simulink model "ClosedLoopSys"  (R2025b)
settings: Solver=ode4  StartTime=0.00  StopTime=10  FixedStep=T  RelTol=1e-5  EnableMultiTasking=on
undefined symbols (not defined in the file or in its folder): amp_sat_l, amp_sat_u, DAC_lim_l, DAC_lim_u, Discrete, g, Je, Jp, Jt, k_d, k_fan, k_N, k_s, l, l1, l2, l3, m1, m2, N, nu, nx, Q, q, QN, sys_fan, T, T_mpc, Time, U_e, x0, xfe
libraries: ctrlSharedLib x1
settings Model: Creator=bjones  LastModifiedBy=leeta
settings SolverCC: AlgebraicLoopSolver=TrustRegion
settings DataIOCC: SaveFormat=Array  SignalLoggingSaveFormat=ModelDataLogs  ReturnWorkspaceOutputs=off
settings OptimizationCC: BlockReduction=off  BooleanDataType=off  ExpressionDepthLimit=2147483647.0  LifeSpan=inf
settings DebuggingCC: SaveWithParameterizedLinksMsg=none  MergeDetectMultiDrivingBlocksExec=none  SignalResolutionControl=TryResolveAllWithWarning  MultiTaskDSMMsg=warning  MultiTaskCondExecSysMsg=none  FcnCallInpInsideContextMsg=warning  UnconnectedInputMsg=warning  UnconnectedOutputMsg=warning  UnconnectedLineMsg=warning  StateNameClashWarn=warning  SFUnexpectedBacktrackingDiag=warning  SFNoUnconditionalDefaultTransitionDiag=warning  SFExecutionAtInitializationDiag=none  ArithmeticOperatorsInVariantConditions=warning
settings HardwareCC: ProdBitPerPointer=32.0  ProdBitPerSizeT=32.0  ProdBitPerPtrDiffT=32.0  ProdLargestAtomicFloat=None  ProdIntDivRoundTo=Undefined  ProdEndianess=Unspecified  ProdWordSize=32.0  ProdHWDeviceType=32-bit Generic  TargetUnknown=on
settings ModelReferenceCC: EnableRefExpFcnMdlSchedulingChecks=on  PropagateSignalLabelsOutOfModel=off
settings SFSimCC: SimUseLocalCustomCode=off  CustomCodeUndefinedFunction=UseInterfaceOnly
settings RTWCC: RTWUseLocalCustomCode=off  GPUComputeCapability=3.5
settings CodeAppCC: StateflowObjectComments=on
settings GRTTargetCC: TargetLangStandard=C89/C90 (ANSI)  CombineOutputUpdateFcns=off  GRTInterface=on
settings ConfigComp: CovMetricSettings=dw  CovSaveCumulativeToWorkspaceVar=on  CovSaveSingleToWorkspaceVar=on  CovExternalEMLEnable=off  CovSFcnEnable=off

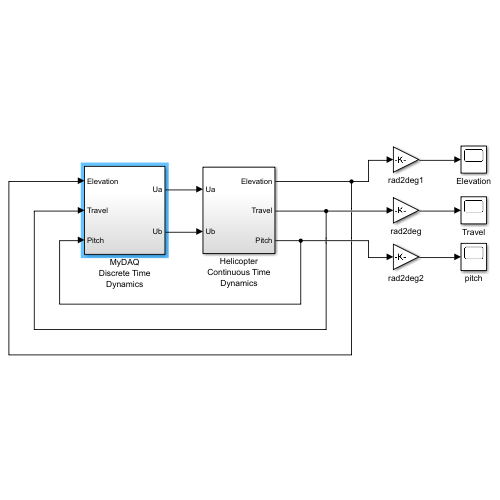
[thumbnail: Simulink's stored preview of the top-level diagram]
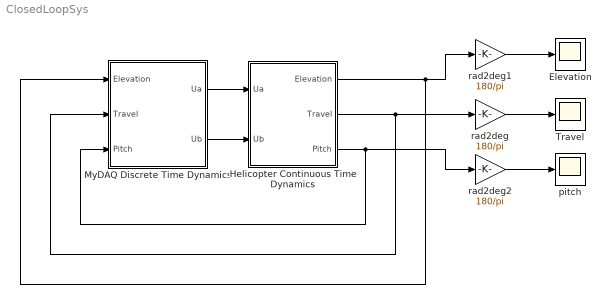
== system ClosedLoopSys ==
  Elevation : Scope
      settings: TimeSpan=60  ActiveDisplayYMinimum=-50  ActiveDisplayYMaximum=30  DataLoggingVariableName=elev
  Helicopter Continuous Time Dynamics : Subsystem
  MyDAQ Discrete Time Dynamics : Subsystem
  Travel : Scope
      settings: TimeSpan=60  ActiveDisplayYMinimum=-150  ActiveDisplayYMaximum=300  DataLoggingVariableName=trav
  pitch : Scope
      settings: TimeSpan=60  ActiveDisplayYMinimum=-25  ActiveDisplayYMaximum=20  DataLoggingVariableName=pitch
  rad2deg : Gain  Gain=180/pi  SaturateOnIntegerOverflow=on  OutDataTypeStr=Inherit: Same as input  ParamDataTypeStr=Inherit: Same as input
  rad2deg1 : Gain  Gain=180/pi  SaturateOnIntegerOverflow=on  OutDataTypeStr=Inherit: Same as input  ParamDataTypeStr=Inherit: Same as input
  rad2deg2 : Gain  Gain=180/pi  SaturateOnIntegerOverflow=on  OutDataTypeStr=Inherit: Same as input  ParamDataTypeStr=Inherit: Same as input
  wires:
  rad2deg/1 -> Travel/1
  rad2deg1/1 -> Elevation/1
  Helicopter Continuous Time Dynamics/2(Travel) -> MyDAQ Discrete Time Dynamics/2(Travel), rad2deg/1
  Helicopter Continuous Time Dynamics/1(Elevation) -> rad2deg1/1, MyDAQ Discrete Time Dynamics/1(Elevation)
  rad2deg2/1 -> pitch/1
  Helicopter Continuous Time Dynamics/3(Pitch) -> rad2deg2/1, MyDAQ Discrete Time Dynamics/3(Pitch)
  MyDAQ Discrete Time Dynamics/1(Ua) -> Helicopter Continuous Time Dynamics/1(Ua)
  MyDAQ Discrete Time Dynamics/2(Ub) -> Helicopter Continuous Time Dynamics/2(Ub)

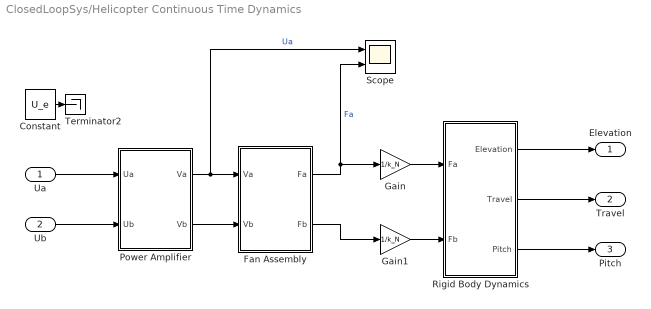
== system ClosedLoopSys/Helicopter Continuous Time Dynamics ==
  Ua : Inport
  Ub : Inport  Port=2
  Constant : Constant  Value=U_e
  Fan Assembly : Subsystem
  Gain : Gain  Gain=1/k_N
  Gain1 : Gain  Gain=1/k_N
  Power Amplifier : Subsystem
  Rigid Body Dynamics : Subsystem
  Scope : Scope  NumInputPorts=2
      settings: ActiveDisplayYMinimum=-1.0960612962914624  ActiveDisplayYMaximum=9.9757218399878962  DataLoggingVariableName=ScopeData5
  Terminator2 : Terminator
  Elevation : Outport
  Travel : Outport  Port=2
  Pitch : Outport  Port=3
  wires:
  Power Amplifier/1(Va) -> Scope/1, Fan Assembly/1(Va)  "Ua"
  Power Amplifier/2(Vb) -> Fan Assembly/2(Vb)
  Rigid Body Dynamics/1(Elevation) -> Elevation/1
  Rigid Body Dynamics/3(Pitch) -> Pitch/1
  Fan Assembly/2(Fb) -> Gain1/1
  Rigid Body Dynamics/2(Travel) -> Travel/1
  Fan Assembly/1(Fa) -> Scope/2, Gain/1  "Fa"
  Ub/1 -> Power Amplifier/2(Ub)
  Constant/1 -> Terminator2/1
  Ua/1 -> Power Amplifier/1(Ua)
  Gain/1 -> Rigid Body Dynamics/1(Fa)
  Gain1/1 -> Rigid Body Dynamics/2(Fb)

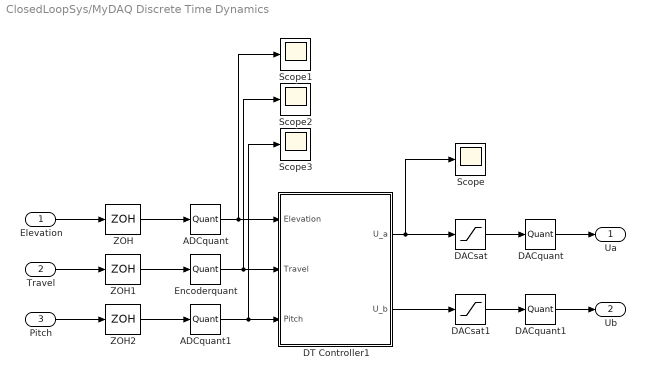
== system ClosedLoopSys/MyDAQ Discrete Time Dynamics ==
  Elevation : Inport
  Travel : Inport  Port=2
  Pitch : Inport  Port=3
  ADCquant : Quantizer  QuantizationInterval=ADC_Vres  SampleTime=T
  ADCquant1 : Quantizer  QuantizationInterval=ADC_Vres  SampleTime=T
  DACquant : Quantizer  QuantizationInterval=DAC_Vres  SampleTime=T
  DACquant1 : Quantizer  QuantizationInterval=DAC_Vres  SampleTime=T
  DACsat : Saturate  UpperLimit=DAC_lim_u  LowerLimit=DAC_lim_l  SampleTime=T
  DACsat1 : Saturate  UpperLimit=DAC_lim_u  LowerLimit=DAC_lim_l  SampleTime=T
  DT Controller1 : Subsystem
  Encoderquant : Quantizer  QuantizationInterval=Encoder_res  SampleTime=T
  Scope{,1..3} (4 alike) : Scope
      Scope settings: ActiveDisplayYMinimum=-1  ActiveDisplayYMaximum=1
      Scope1 settings: ActiveDisplayYMinimum=-0.1017  ActiveDisplayYMaximum=0.78714  DataLoggingVariableName=ScopeData2
      Scope2 settings: ActiveDisplayYMinimum=-1  ActiveDisplayYMaximum=1
      Scope3 settings: ActiveDisplayYMinimum=-1  ActiveDisplayYMaximum=1  DataLoggingVariableName=ScopeData2
  ZOH : ZeroOrderHold  SampleTime=T
  ZOH1 : ZeroOrderHold  SampleTime=T
  ZOH2 : ZeroOrderHold  SampleTime=T
  Ua : Outport
  Ub : Outport  Port=2
  wires:
  Elevation/1 -> ZOH/1
  Travel/1 -> ZOH1/1
  DACquant/1 -> Ua/1
  DACquant1/1 -> Ub/1
  DT Controller1/1(U_a) -> Scope/1, DACsat/1
  DACsat/1 -> DACquant/1
  DT Controller1/2(U_b) -> DACsat1/1
  DACsat1/1 -> DACquant1/1
  ZOH1/1 -> Encoderquant/1
  ZOH/1 -> ADCquant/1
  Pitch/1 -> ZOH2/1
  ZOH2/1 -> ADCquant1/1
  ADCquant/1 -> Scope1/1, DT Controller1/1(Elevation)
  ADCquant1/1 -> Scope3/1, DT Controller1/3(Pitch)
  Encoderquant/1 -> Scope2/1, DT Controller1/2(Travel)

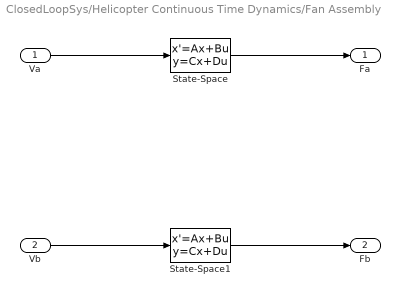
== system ClosedLoopSys/Helicopter Continuous Time Dynamics/Fan Assembly ==
  Va : Inport
  Vb : Inport  Port=2
  State-Space : StateSpace  A=sys_fan.A  B=sys_fan.B  C=sys_fan.C  D=sys_fan.D  InitialCondition=U_e*k_fan
  State-Space1 : StateSpace  A=sys_fan.A  B=sys_fan.B  C=sys_fan.C  D=sys_fan.D  InitialCondition=U_e*k_fan
  Fa : Outport
  Fb : Outport  Port=2
  wires:
  Va/1 -> State-Space/1
  State-Space1/1 -> Fb/1
  Vb/1 -> State-Space1/1
  State-Space/1 -> Fa/1

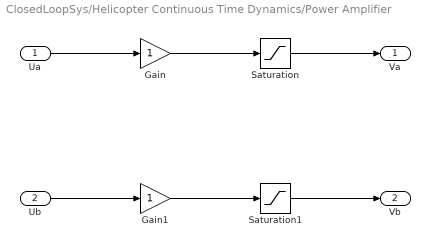
== system ClosedLoopSys/Helicopter Continuous Time Dynamics/Power Amplifier ==
  Ua : Inport
  Ub : Inport  Port=2
  Gain : Gain
  Gain1 : Gain
  Saturation : Saturate  UpperLimit=amp_sat_u  LowerLimit=amp_sat_l
  Saturation1 : Saturate  UpperLimit=amp_sat_u  LowerLimit=amp_sat_l
  Va : Outport
  Vb : Outport  Port=2
  wires:
  Ua/1 -> Gain/1
  Gain/1 -> Saturation/1
  Saturation/1 -> Va/1
  Saturation1/1 -> Vb/1
  Gain1/1 -> Saturation1/1
  Ub/1 -> Gain1/1

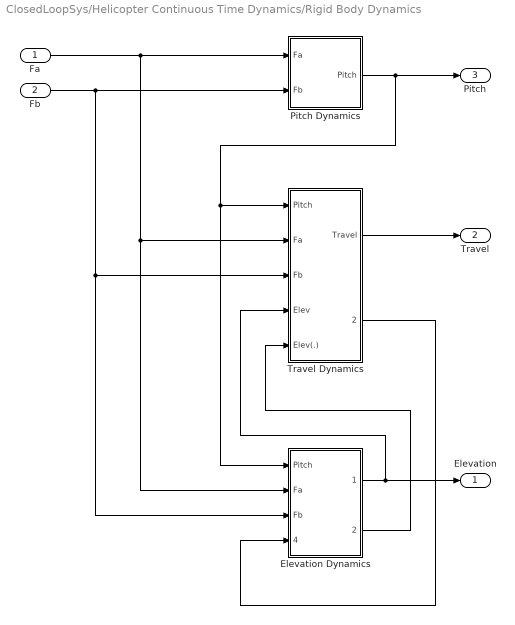
== system ClosedLoopSys/Helicopter Continuous Time Dynamics/Rigid Body Dynamics ==
  Fa : Inport
  Fb : Inport  Port=2
  Elevation Dynamics : Subsystem
  Pitch Dynamics : Subsystem
  Travel Dynamics : Subsystem
  Elevation : Outport
  Travel : Outport  Port=2
  Pitch : Outport  Port=3
  wires:
  Fa/1 -> Pitch Dynamics/1(Fa), Travel Dynamics/2(Fa), Elevation Dynamics/2(Fa)
  Fb/1 -> Pitch Dynamics/2(Fb), Elevation Dynamics/3(Fb), Travel Dynamics/3(Fb)
  Travel Dynamics/1(Travel) -> Travel/1
  Elevation Dynamics/1(Elevation) -> Elevation/1, Travel Dynamics/4(Elev)
  Pitch Dynamics/1(Pitch) -> Travel Dynamics/1(Pitch), Elevation Dynamics/1(Pitch), Pitch/1
  Travel Dynamics/2(Travel(.)) -> Elevation Dynamics/4(Travel(.))
  Elevation Dynamics/2(Elevation(.)) -> Travel Dynamics/5(Elev(.))

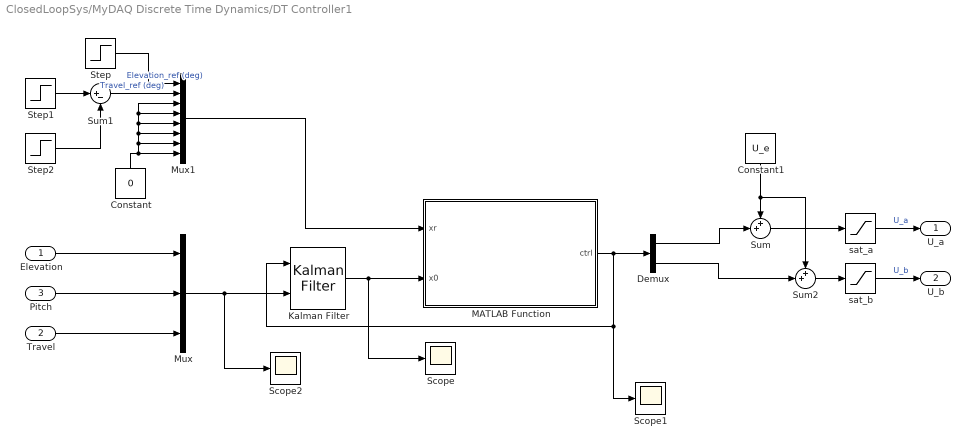
== system ClosedLoopSys/MyDAQ Discrete Time Dynamics/DT Controller1 ==
  Elevation : Inport
  Travel : Inport  Port=2
  Pitch : Inport  Port=3
  Constant : Constant  Value=0
  Constant1 : Constant  Value=U_e
  Demux : Demux  Outputs=2
  Kalman Filter : ctrlSharedLib/Kalman Filter  TimeDomain=Discrete-Time  UseCurrentEstimator=on  ModelSource=LTI State-Space Variable  ModelSourceVariable=sysdt_comb  A=0.95  B=1  C=1  D=0  NumberOfStates=1  NumberOfInputs=1  NumberOfOutputs=1  InitialEstimateSource=Dialog  X0=x0  P0=10  UseK=off  UseGH=off  NumberOfProcessNoiseInputs=1  G=1  TimeInvariantG=on  H=0  TimeInvariantH=on  Q=0.05  TimeInvariantQ=on  R=1  TimeInvariantR=on  N=0  TimeInvariantN=on  AddInputPort=on  AddEnablePort=off  OutputEstimatedY=off  OutputP=off  Ts=-1
  MATLAB Function : MATLAB Function  TreatAsAtomicUnit=on
  Mux : Mux  Inputs=3
  Mux1 : Mux  Inputs=8
  Scope : Scope
      settings: ActiveDisplayYMinimum=-2.4396283803217269  ActiveDisplayYMaximum=1.6155430663981798  DataLoggingVariableName=ScopeData3
  Scope1 : Scope
      settings: ActiveDisplayYMinimum=-1.19057  ActiveDisplayYMaximum=4.48934  DataLoggingVariableName=ScopeData4
  Scope2 : Scope
      settings: ActiveDisplayYMinimum=-0.1017  ActiveDisplayYMaximum=0.78714  DataLoggingVariableName=ScopeData3
  Step : Step  Time=0  Before=x0(1)  After=0  SampleTime=T_mpc
  Step1 : Step  Time=x0(2)  After=0  SampleTime=T_mpc
  Step2 : Step  Time=0  Before=x0(3)  After=0  SampleTime=T_mpc
  Sum : Sum  Inputs=++|
  Sum1 : Sum  Inputs=|+-
  Sum2 : Sum  Inputs=++|
  sat_a : Saturate  UpperLimit=DAC_lim_u  LowerLimit=DAC_lim_l
  sat_b : Saturate  UpperLimit=DAC_lim_u  LowerLimit=DAC_lim_l
  U_a : Outport
  U_b : Outport  Port=2
  wires:
  Step1/1 -> Sum1/1
  Step2/1 -> Sum1/2
  sat_b/1 -> U_b/1  "U_b"
  sat_a/1 -> U_a/1  "U_a"
  Step/1 -> Mux1/1  "Elevation_ref (deg)"
  Sum1/1 -> Mux1/2  "Travel_ref (deg)"
  Elevation/1 -> Mux/1
  Pitch/1 -> Mux/2
  Travel/1 -> Mux/3
  Mux/1 -> Scope2/1, Kalman Filter/2
  Kalman Filter/1 -> Scope/1, MATLAB Function/2(x0)
  MATLAB Function/1(ctrl) -> Scope1/1, Kalman Filter/1, Demux/1
  Constant/1 -> Mux1/8, Mux1/6, Mux1/4, Mux1/3, Mux1/5, Mux1/7
  Mux1/1 -> MATLAB Function/1(xr)
  Demux/1 -> Sum/2
  Demux/2 -> Sum2/2
  Sum/1 -> sat_a/1
  Sum2/1 -> sat_b/1
  Constant1/1 -> Sum2/1, Sum/1

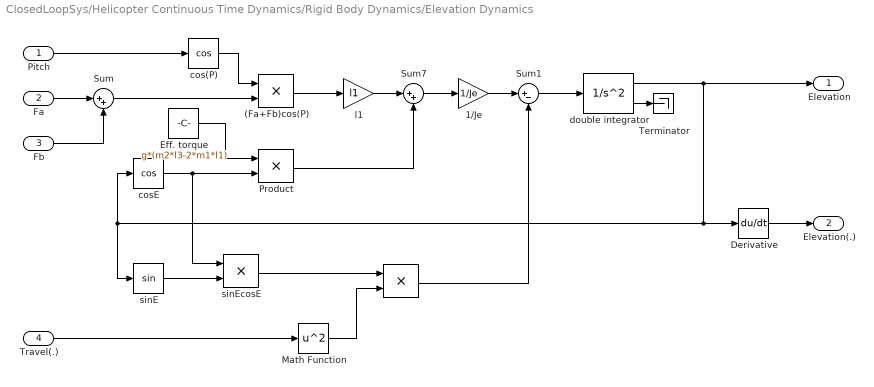
== system ClosedLoopSys/Helicopter Continuous Time Dynamics/Rigid Body Dynamics/Elevation Dynamics ==
  Pitch : Inport
  Fa : Inport  Port=2
  Fb : Inport  Port=3
  Travel(.) : Inport  Port=4
  " " : Product  InputSameDT=on  RndMeth=Zero  SaturateOnIntegerOverflow=on  OutDataTypeStr=Inherit: Same as first input
  (Fa+Fb)cos(P) : Product  InputSameDT=on  RndMeth=Zero  SaturateOnIntegerOverflow=on  OutDataTypeStr=Inherit: Same as first input
  1/Je : Gain  Gain=1/Je  SaturateOnIntegerOverflow=on  OutDataTypeStr=Inherit: Same as input  ParamDataTypeStr=Inherit: Same as input
  Derivative : Derivative
  Eff. torque : Constant  Value=g*(m2*l3-2*m1*l1)
  Math Function : Math  Operator=square  SignedPower=on
  Product : Product  InputSameDT=on  RndMeth=Zero  SaturateOnIntegerOverflow=on  OutDataTypeStr=Inherit: Same as first input
  Sum : Sum  Inputs=|++  InputSameDT=on  SaturateOnIntegerOverflow=on  OutDataTypeStr=Inherit: Same as first input
  Sum1 : Sum  Inputs=|+-  InputSameDT=on  SaturateOnIntegerOverflow=on  OutDataTypeStr=Inherit: Same as first input
  Sum7 : Sum  Inputs=|++  InputSameDT=on  SaturateOnIntegerOverflow=on  OutDataTypeStr=Inherit: Same as first input
  Terminator : Terminator
  cos(P) : Trigonometry  Operator=cos
  cosE : Trigonometry  Operator=cos
  double integrator : SecondOrderIntegrator  ICX=x0(3)  LimitX=on  UpperLimitX=e_lim_u  LowerLimitX=e_lim_l  LimitDXDT=on  UpperLimitDXDT=2*pi  LowerLimitDXDT=-2*pi
  l1 : Gain  Gain=l1  SaturateOnIntegerOverflow=on  OutDataTypeStr=Inherit: Same as input  ParamDataTypeStr=Inherit: Same as input
  sinE : Trigonometry
  sinEcosE : Product  InputSameDT=on  RndMeth=Zero  SaturateOnIntegerOverflow=on  OutDataTypeStr=Inherit: Same as first input
  Elevation : Outport
  Elevation(.) : Outport  Port=2
  wires:
  double integrator/1 -> Elevation/1, sinE/1, cosE/1, Derivative/1
  Derivative/1 -> Elevation(.)/1
  double integrator/2 -> Terminator/1
  Pitch/1 -> cos(P)/1
  Fa/1 -> Sum/1
  Fb/1 -> Sum/2
  cos(P)/1 -> (Fa+Fb)cos(P)/1
  Sum/1 -> (Fa+Fb)cos(P)/2
  (Fa+Fb)cos(P)/1 -> l1/1
  l1/1 -> Sum7/1
  Sum7/1 -> 1/Je/1
  1/Je/1 -> Sum1/1
  Sum1/1 -> double integrator/1
  Travel(.)/1 -> Math Function/1
  Eff. torque/1 -> Product/1
  cosE/1 -> sinEcosE/1, Product/2
  sinE/1 -> sinEcosE/2
  sinEcosE/1 -> " "/1
  Math Function/1 -> " "/2
  Product/1 -> Sum7/2
  " "/1 -> Sum1/2

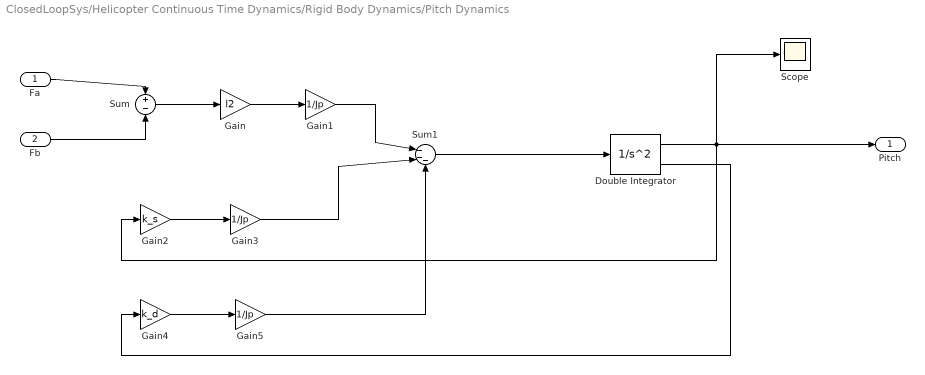
== system ClosedLoopSys/Helicopter Continuous Time Dynamics/Rigid Body Dynamics/Pitch Dynamics ==
  Fa : Inport
  Fb : Inport  Port=2
  Double Integrator : SecondOrderIntegrator  ICX=x0(1)  LimitX=on  UpperLimitX=p_lim_u  LowerLimitX=p_lim_l
  Gain : Gain  Gain=l2
  Gain1 : Gain  Gain=1/Jp
  Gain2 : Gain  Gain=k_s
  Gain3 : Gain  Gain=1/Jp
  Gain4 : Gain  Gain=k_d
  Gain5 : Gain  Gain=1/Jp
  Scope : Scope
      settings: ActiveDisplayYMinimum=-1  ActiveDisplayYMaximum=1  DataLoggingVariableName=ScopeData2
  Sum : Sum  Inputs=+-
  Sum1 : Sum  Inputs=|---
  Pitch : Outport
  wires:
  Fa/1 -> Sum/1
  Gain4/1 -> Gain5/1
  Sum1/1 -> Double Integrator/1
  Fb/1 -> Sum/2
  Gain1/1 -> Sum1/1
  Gain2/1 -> Gain3/1
  Gain5/1 -> Sum1/3
  Double Integrator/2 -> Gain4/1
  Gain/1 -> Gain1/1
  Sum/1 -> Gain/1
  Gain3/1 -> Sum1/2
  Double Integrator/1 -> Pitch/1, Scope/1, Gain2/1

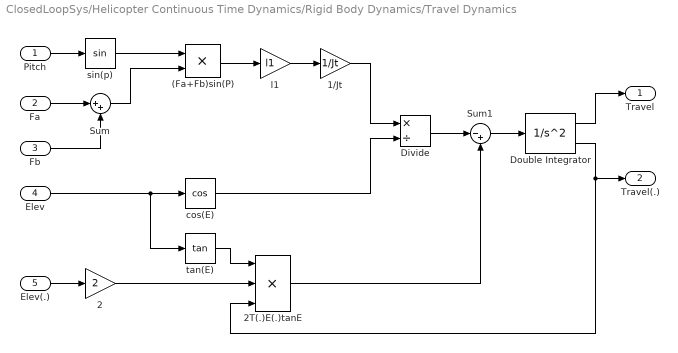
== system ClosedLoopSys/Helicopter Continuous Time Dynamics/Rigid Body Dynamics/Travel Dynamics ==
  Pitch : Inport
  Fa : Inport  Port=2
  Fb : Inport  Port=3
  Elev : Inport  Port=4
  Elev(.) : Inport  Port=5
  (Fa+Fb)sin(P) : Product  InputSameDT=on  RndMeth=Zero  SaturateOnIntegerOverflow=on  OutDataTypeStr=Inherit: Same as first input
  1/Jt : Gain  Gain=1/Jt  SaturateOnIntegerOverflow=on  OutDataTypeStr=Inherit: Same as input  ParamDataTypeStr=Inherit: Same as input
  2 : Gain  Gain=2  SaturateOnIntegerOverflow=on  OutDataTypeStr=Inherit: Same as input  ParamDataTypeStr=Inherit: Same as input
  2T(.)E(.)tanE : Product  Inputs=3  InputSameDT=on  RndMeth=Zero  SaturateOnIntegerOverflow=on  OutDataTypeStr=Inherit: Same as first input
  Divide : Product  Inputs=*/
  Double Integrator : SecondOrderIntegrator  ICX=x0(2)  UpperLimitX=1  LowerLimitX=0  LimitDXDT=on  UpperLimitDXDT=2  LowerLimitDXDT=-2
  Sum : Sum  Inputs=|++  InputSameDT=on  SaturateOnIntegerOverflow=on  OutDataTypeStr=Inherit: Same as first input
  Sum1 : Sum  Inputs=|-+  InputSameDT=on  SaturateOnIntegerOverflow=on  OutDataTypeStr=Inherit: Same as first input
  cos(E) : Trigonometry  Operator=cos
  l1 : Gain  Gain=l1  SaturateOnIntegerOverflow=on  OutDataTypeStr=Inherit: Same as input  ParamDataTypeStr=Inherit: Same as input
  sin(p) : Trigonometry
  tan(E) : Trigonometry  Operator=tan
  Travel : Outport
  Travel(.) : Outport  Port=2
  wires:
  Double Integrator/1 -> Travel/1
  sin(p)/1 -> (Fa+Fb)sin(P)/1
  (Fa+Fb)sin(P)/1 -> l1/1
  Pitch/1 -> sin(p)/1
  Fa/1 -> Sum/1
  Fb/1 -> Sum/2
  Sum/1 -> (Fa+Fb)sin(P)/2
  l1/1 -> 1/Jt/1
  Elev/1 -> cos(E)/1, tan(E)/1
  1/Jt/1 -> Divide/1
  cos(E)/1 -> Divide/2
  Double Integrator/2 -> Travel(.)/1, 2T(.)E(.)tanE/3
  tan(E)/1 -> 2T(.)E(.)tanE/1
  Elev(.)/1 -> 2/1
  2/1 -> 2T(.)E(.)tanE/2
  Divide/1 -> Sum1/1
  Sum1/1 -> Double Integrator/1
  2T(.)E(.)tanE/1 -> Sum1/2

== matlab function ClosedLoopSys/MyDAQ Discrete Time Dynamics/DT Controller1/MATLAB Function ==
  data: xr input double size=nx; x0 input double size=nx; ctrl output double size=nu; l parameter; u parameter; q parameter; Q parameter; QN parameter; nx parameter; nu parameter; N parameter; xfe parameter; U_e parameter double size=1
function ctrl = mpc_step(xr, x0, l, u, q, Q, QN, nx, nu, N, xfe, U_e)

    coder.extrinsic('emosqp')
    % Update OSQP problem
    % Update initial state

    l(1:nx) = -x0;
    u(1:nx) = -x0;
    % l(1:nx) = -(x0-xfe);
    % u(1:nx) = -(x0-xfe);

    % Update cost for variable xr
    q = [repmat(-Q*xr, N, 1); -QN*xr; zeros(N*nu, 1)];

    emosqp('update_bounds', l, u);
    emosqp('update_lin_cost', q);

    [x, ~, ~, ~, ~] = emosqp('solve'); 

    ctrl = x((N+1)*nx+1:(N+1)*nx+nu);
    % ctrl(1) = ctrl(1) + U_e;
    % ctrl(2) = ctrl(2) + U_e;
end
